simulink model "reg_4_model"  (R2019b)
settings: Solver=VariableStepAuto  StartTime=reg4.ti  StopTime=inf  MaxStep=1e-4  RelTol=1e-9
undefined symbols (not defined in the file): reg4
settings Model: Creator=Charlie  LastModifiedBy=nash

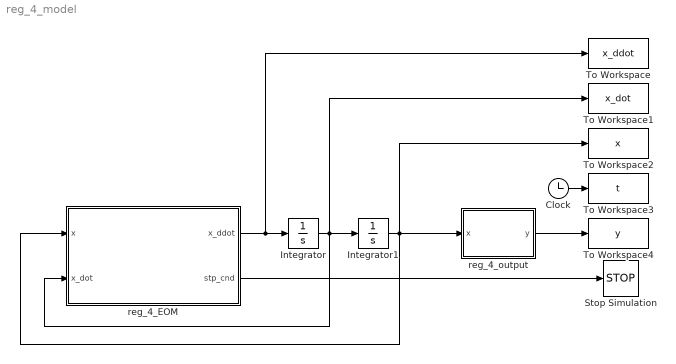
== system reg_4_model ==
  Clock : Clock
  Integrator : Integrator  InitialCondition=reg4.xi_dot
  Integrator1 : Integrator  InitialCondition=reg4.xi
  Stop Simulation : Stop
  To Workspace : ToWorkspace  VariableName=x_ddot  SampleTime=-1
  To Workspace1 : ToWorkspace  VariableName=x_dot  SampleTime=-1
  To Workspace2 : ToWorkspace  VariableName=x  SampleTime=-1
  To Workspace3 : ToWorkspace  VariableName=t  SampleTime=-1
  To Workspace4 : ToWorkspace  VariableName=y  SampleTime=-1
  reg_4_EOM : MATLAB Function  TreatAsAtomicUnit=on
  reg_4_output : MATLAB Function  TreatAsAtomicUnit=on
  wires:
  reg_4_EOM/1(x_ddot) -> To Workspace/1, Integrator/1
  reg_4_output/1(y) -> To Workspace4/1
  Clock/1 -> To Workspace3/1
  Integrator1/1 -> To Workspace2/1, reg_4_EOM/1(x), reg_4_output/1(x)
  reg_4_EOM/2(stp_cnd) -> Stop Simulation/1
  Integrator/1 -> To Workspace1/1, reg_4_EOM/2(x_dot), Integrator1/1

== matlab function reg_4_model/reg_4_output ==
  data: x input; y output; P parameter
%% Regime 4 output equations
%
% This function is responsible for converting the state variables in x to
% the x- and y-coordinates for each point in the mechanism.
%
% This function takes in the following parameters
%   x           The state vector representing the x- and y- coordinates of
%               the projectile.
%   P           A MATLAB struct containing all of the constant parameters
% 
% The function returns the following parameters
%   y           The output vector containing the x- and y- coordinates for
%               each point in the mechanism
%
function y  = reg_4_output(x, P)

y = zeros(14,1);

% Point A
y(1)  = 0;                                              % <------
y(2)  = 0;                                              % <------

% Point B
y(3)  = 0;                                              % <------
y(4)  = 0;                                              % <------

% Point C
y(7)  = 0;                                              % <------
y(8)  = 0;                                              % <------

% Point D
y(5)  = 0;                                              % <------
y(6)  = 0;                                              % <------

% Point E
y(9)  = 0;                                              % <------
y(10) = 0;                                              % <------

% Point F
y(11) = 0;                                              % <------
y(12) = 0;                                              % <------

% Point G
y(13) = 0;                                              % <------
y(14) = 0;                                              % <------

== matlab function reg_4_model/reg_4_EOM ==
  data: x input; x_dot input; x_ddot output; stp_cnd output; P parameter
% Regime 4 equations of motion
%
% This function is responsible for determining the time rate-of-change of
% the state vector representing the location of the projectile during
% Regime 4.
%
% Regime 4 is the flying regime in which the projectile is flying through
% the air.
%
% This function takes in the following parameters
%   x           The state vector representing the x and y displacement of
%               the projectile.
%   x_dot       The velocity vector representing the x and y velocity of
%               the projectile.
%   P           A MATLAB struct containing all of the constant parameters
% 
% The function returns the following parameters
%   x_ddot      The acceleration vector representing the x and y
%               acceleration of the projectile.
%   stp_cnd     The stop condition for the simulation. Turns true when
%               the projectile hits the ground.
%
function [x_ddot, stp_cnd] = reg_4_EOM(x, x_dot, P)

% For this regime the acceleration equations are nearly trivial. The
% projectile is simply a particle acted upon by gravity alone.
x_ddot = [ 0
           P.g ];

% The stop condition becomes true when the vertical displacement of point E
% become negative indicating that the projectile has hit the ground.
stp_cnd = true;
